simulink model "d_flip_flop"  (R2018a)
settings: Solver=VariableStepAuto  StartTime=0.0  StopTime=10.0  RelTol=1e-3
settings Model: Creator=Edoardo Debenedetti  LastModifiedBy=Edoardo Debenedetti

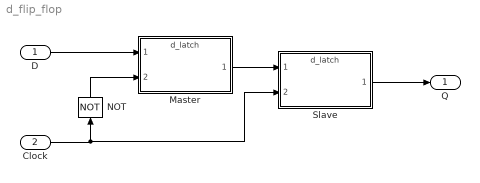
== system d_flip_flop ==
  D : Inport
  Clock : Inport  Port=2
  Master : ModelReference  ModelNameDialog=d_latch  SimulationMode=Normal  ModelReferenceVersion=1.1
  NOT : Logic  Operator=NOT  IconShape=distinctive  AllPortsSameDT=off  OutDataTypeStr=boolean
  Slave : ModelReference  ModelNameDialog=d_latch  SimulationMode=Normal  ModelReferenceVersion=1.1
  Q : Outport
  wires:
  Master/1 -> Slave/1
  D/1 -> Master/1
  Clock/1 -> Slave/2, NOT/1
  NOT/1 -> Master/2
  Slave/1 -> Q/1
